simulink model "untitled"  (R2025b)
settings: Solver=VariableStepAuto  StartTime=0.0  StopTime=2  RelTol=1e-3
undefined symbols (not defined in the file or in its folder): designMultirateFIR
libraries: dspxfrm3 x2, dspfdesign x1, dspmlti4 x1
settings Model: Creator=janek  LastModifiedBy=janek

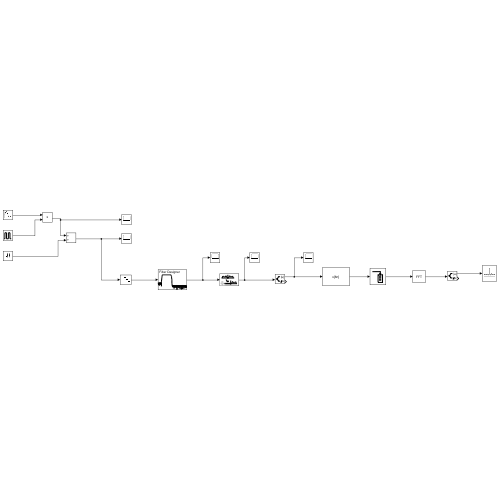
[thumbnail: Simulink's stored preview of the top-level diagram]
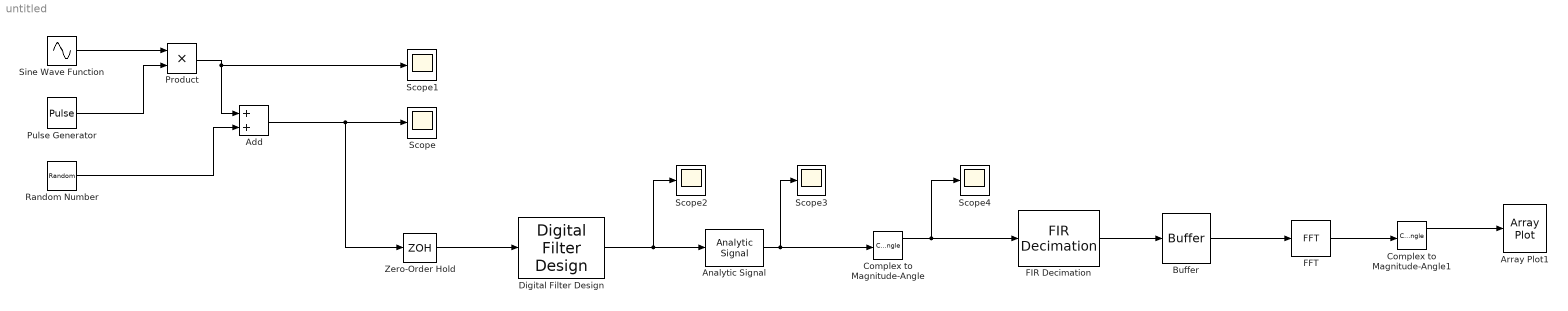
== system untitled ==
  Add : Sum
  Analytic Signal : dspxfrm3/Analytic Signal  N=100  InputProcessing=Columns as channels (frame based)
  Array Plot1 : ArrayPlot  WindowPosition=[880.000000,470.000000,800.000000,500.000000,]  ScopeFrameLocation=window  MaximizeAxes=Off  YLimits=[-32.50163548924309 26.00357890919143]
  Buffer : Buffer  N=1024  OutputFrames=off
  Complex to Magnitude-Angle : ComplexToMagnitudeAngle
  Complex to Magnitude-Angle1 : ComplexToMagnitudeAngle
  Digital Filter Design : dspfdesign/Digital Filter Design  mwdsp_browser_bugfix_var=off
  FFT : dspxfrm3/FFT  FFTImplementation=Auto  CompMethod=Table lookup  TableOpt=NEW  TableOptActive=Speed  BitRevOrder=off  Normalize=off  InheritFFTLength=on  FFTLength=64  WrapInput=on  roundingMode=Ceiling  overflowMode=off  firstCoeffDataTypeStr=Inherit: Same word length as input  firstCoeffLastDataTypeStr=Inherit: Same word length as input  outputMin=[]  outputMax=[]
  FIR Decimation : dspmlti4/FIR Decimation  FilterSource=Auto  h=designMultirateFIR(1,2)  D=8  filtStruct=Direct form  FilterObject=FDECIM  InputProcessing=Columns as channels (frame based)  framing=Allow multirate processing  AllowArbitraryInputLength=off  inputOffset=0  outputBufInitCond=0  roundingMode=Floor  overflowMode=off  firstCoeffDataTypeStr=Inherit: Same word length as input  firstCoeffMin=[]  firstCoeffMax=[]  firstCoeffLastDataTypeStr=Inherit: Same word length as input  outputDataTypeStr=Inherit: Same as accumulator  outputMin=[]  outputMax=[]  outputLastDataTypeStr=Inherit: Same as accumulator
  Product : Product
  Pulse Generator : DiscretePulseGenerator  PulseType=Time based  Period=0.01  PulseWidth=2
  Random Number : RandomNumber  Variance=0.2  SampleTime=1/26770
  Scope{,1..4} (5 alike) : Scope
      Scope settings: ActiveDisplayYMinimum=-3.0855531603587423  ActiveDisplayYMaximum=3.7589820192134162
      Scope1 settings: ActiveDisplayYMinimum=-2.0822795442827871  ActiveDisplayYMaximum=2.4303516707747135
      Scope2 settings: ActiveDisplayYMinimum=-2.0822795442827871  ActiveDisplayYMaximum=2.4303516707747135  DataLoggingVariableName=ScopeData2
      Scope3 settings: ActiveDisplayYMinimum=-2.0822795442827871  ActiveDisplayYMaximum=2.4303516707747135  DataLoggingVariableName=ScopeData3
      Scope4 settings: ActiveDisplayYMinimum=-2.0822795442827871  ActiveDisplayYMaximum=2.4303516707747135  DataLoggingVariableName=ScopeData4
  Sine Wave Function : Sin  Frequency=25133  SampleTime=0
  Zero-Order Hold : ZeroOrderHold  SampleTime=1/26770
  wires:
  Sine Wave Function/1 -> Product/1
  Pulse Generator/1 -> Product/2
  Product/1 -> Scope1/1, Add/1
  Random Number/1 -> Add/2
  Add/1 -> Zero-Order Hold/1, Scope/1
  Zero-Order Hold/1 -> Digital Filter Design/1
  Digital Filter Design/1 -> Scope2/1, Analytic Signal/1
  Analytic Signal/1 -> Scope3/1, Complex to Magnitude-Angle/1
  Complex to Magnitude-Angle/1 -> FIR Decimation/1, Scope4/1
  Buffer/1 -> FFT/1
  FFT/1 -> Complex to Magnitude-Angle1/1
  Complex to Magnitude-Angle1/1 -> Array Plot1/1
  FIR Decimation/1 -> Buffer/1
